simulink model "robot1v2"  (R2015a)
settings: Solver=FixedStepDiscrete  StartTime=0.0  StopTime=5  FixedStep=0.05  RelTol=1e-3
settings Model: ExtModeTrigDuration=2  Creator=Antivariant  LastModifiedBy=Antivariant
settings SolverCC: AutoInsertRateTranBlk=on
settings OptimizationCC: OptimizeModelRefInitCode=on  LifeSpan=1
settings DebuggingCC: UnderspecifiedInitializationDetection=Classic  MergeDetectMultiDrivingBlocksExec=none
settings HardwareCC: ProdBitPerInt=16  ProdBitPerPointer=8  ProdIntDivRoundTo=Zero  ProdEndianess=LittleEndian  ProdWordSize=8  ProdHWDeviceType=Atmel->AVR
settings RTWCC: SystemTargetFile=realtime.tlc  GenerateMakefile=off  TemplateMakefile=realtime.tmf  Description=Run on Target Hardware  RTWVerbose=off
settings ERTTargetCC: CombineOutputUpdateFcns=off  ExtModeTransport=3  ExtModeMexFile=ext_serial_win32_comm_rtt  ExtModeMexArgs=0 1 9600  ERTSrcFileBannerTemplate=realtime_code_template.cgt  ERTHdrFileBannerTemplate=realtime_code_template.cgt  ERTDataSrcFileTemplate=realtime_code_template.cgt  ERTDataHdrFileTemplate=realtime_code_template.cgt  ERTCustomFileTemplate=realtime_file_process.tlc

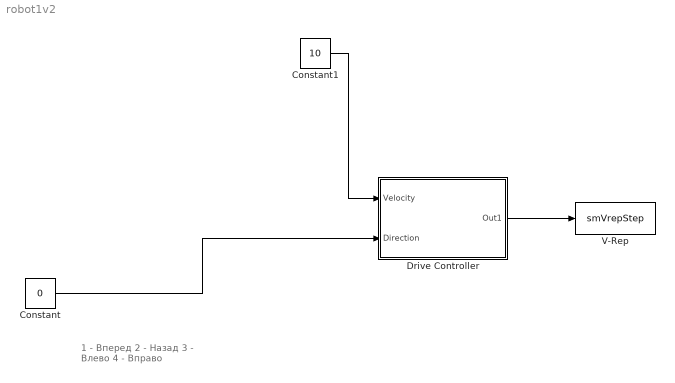
== system robot1v2 ==
  note: 1 - Вперед
      | 2 - Назад
      | 3 - Влево
      | 4 - Вправо
  Constant : Constant  Value=0  OutDataTypeStr=int8
  Constant1 : Constant  Value=10
  Drive Controller : Subsystem
      mask Display:
      | image('wheel.jpg')
      | port_label('input',1,'Velovity')
      | port_label('input',2,'Direction')
  V-Rep : M-S-Function  FunctionName=smVrepStep  Parameters=addr,port  mask{addr='127.0.0.1', port=19997}
      mask Display:
      | port_label('input',1,'in')
      | disp('V-Rep Step')
  wires:
  Constant1/1 -> Drive Controller/1(Velocity)
  Constant/1 -> Drive Controller/2(Direction)
  Drive Controller/1(Out1) -> V-Rep/1

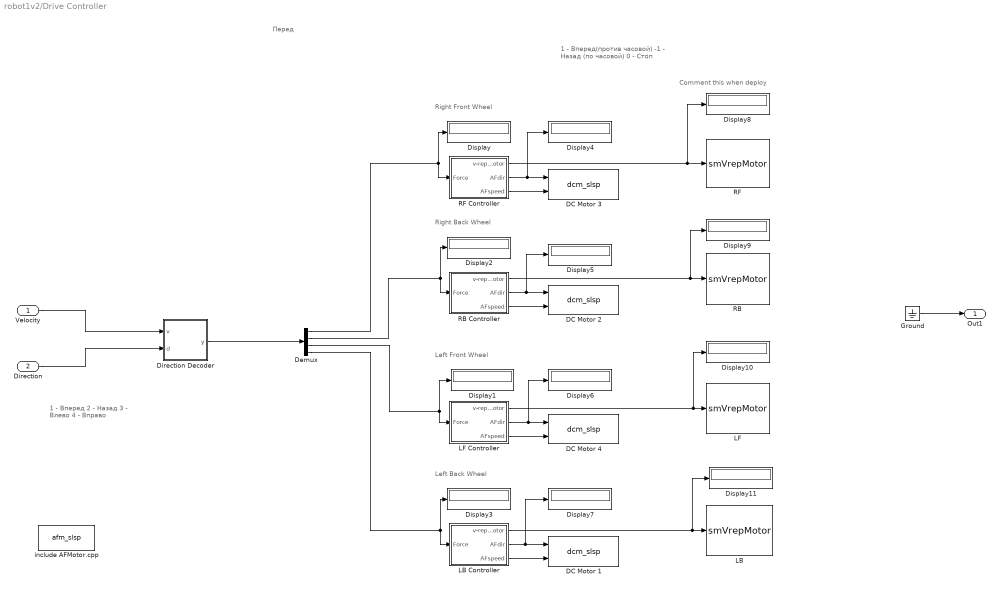
== system robot1v2/Drive Controller ==
  note: Перед
  note: 1 - Вперед
      | 2 - Назад
      | 3 - Влево
      | 4 - Вправо
  note: 1 - Вперед(против часовой)
      | -1 - Назад (по часовой)
      | 0 - Стоп
  note: Comment this when deploy
  note: Right Front Wheel
  note: Left Front Wheel
  note: Right Back Wheel
  note: Left Back Wheel
  Velocity : Inport
  Direction : Inport  Port=2
  DC Motor 1 : S-Function  InitFcn=try, set_param(gcb,'FunctionName','dcm_slsp'), end  FunctionName=dcm_slsp  Parameters=uint8(1)  SFunctionModules=dcm_slsp_wrapper  mask(S-Function Builder){}
      mask init:
      | val = [[.9  0.75 0.75 1 1 .9 .9 1]',[1 1 0.75 0.75 .9 .9 1 .9]'];try , sys = get_param(gcb,'SfunBuilderFcnName');if isempty(sys), sys = get_param(gcb,'FunctionName'); end,catch, sys = get_param(gcb,'FunctionName'); end
      settings: CopyFcn=set_param(gcbh,'LinkStatus','none')  PreSaveFcn=try, set_param(gcb,'FunctionName','dcm_slsp'), end  OpenFcn=sfunctionwizard(gcbh)
      mask Display: plot(val(:,1),val(:,2)),disp(sys), port_label('input',1,'dir'), port_label('input',2,'spd')
  DC Motor 2 : S-Function  InitFcn=try, set_param(gcb,'FunctionName','dcm_slsp'), end  FunctionName=dcm_slsp  Parameters=uint8(2)  SFunctionModules=dcm_slsp_wrapper  mask(S-Function Builder){}
      mask init: same as robot1v2/Drive Controller/DC Motor 1
      settings: CopyFcn=set_param(gcbh,'LinkStatus','none')  PreSaveFcn=try, set_param(gcb,'FunctionName','dcm_slsp'), end  OpenFcn=sfunctionwizard(gcbh)
      mask Display: plot(val(:,1),val(:,2)),disp(sys), port_label('input',1,'dir'), port_label('input',2,'spd')
  DC Motor 3 : S-Function  InitFcn=try, set_param(gcb,'FunctionName','dcm_slsp'), end  FunctionName=dcm_slsp  Parameters=uint8(3)  SFunctionModules=dcm_slsp_wrapper  mask(S-Function Builder){}
      mask init: same as robot1v2/Drive Controller/DC Motor 1
      settings: CopyFcn=set_param(gcbh,'LinkStatus','none')  PreSaveFcn=try, set_param(gcb,'FunctionName','dcm_slsp'), end  OpenFcn=sfunctionwizard(gcbh)
      mask Display: plot(val(:,1),val(:,2)),disp(sys), port_label('input',1,'dir'), port_label('input',2,'spd')
  DC Motor 4 : S-Function  InitFcn=try, set_param(gcb,'FunctionName','dcm_slsp'), end  FunctionName=dcm_slsp  Parameters=uint8(4)  SFunctionModules=dcm_slsp_wrapper  mask(S-Function Builder){}
      mask init: same as robot1v2/Drive Controller/DC Motor 1
      settings: CopyFcn=set_param(gcbh,'LinkStatus','none')  PreSaveFcn=try, set_param(gcb,'FunctionName','dcm_slsp'), end  OpenFcn=sfunctionwizard(gcbh)
      mask Display: plot(val(:,1),val(:,2)),disp(sys), port_label('input',1,'dir'), port_label('input',2,'spd')
  Demux : Demux
  Direction Decoder : Stateflow chart  TreatAsAtomicUnit=on
  Display{,1..11} (12 alike) : Display
  Ground : Ground
  LB : M-S-Function  FunctionName=smVrepMotor  Parameters=addr, port, jname  mask{addr='127.0.0.1', port=19997, jname='joint_back_left_wheel'}
      mask prompts: addr "V-Rep Server Address"; port "V-Rep Server Port"; jname "Joint name"
      mask Display:
      | image('joint.png')
      | port_label('input',1,'vel')
  LB Controller : Subsystem
  LF : M-S-Function  FunctionName=smVrepMotor  Parameters=addr, port, jname  mask{addr='127.0.0.1', port=19997, jname='joint_front_left_wheel'}
      mask prompts: addr "V-Rep Server Address"; port "V-Rep Server Port"; jname "Joint name"
      mask Display:
      | image('joint.png')
      | port_label('input',1,'vel')
  LF Controller : Subsystem
  RB : M-S-Function  FunctionName=smVrepMotor  Parameters=addr, port, jname  mask{addr='127.0.0.1', port=19997, jname='joint_back_right_wheel'}
      mask prompts: addr "V-Rep Server Address"; port "V-Rep Server Port"; jname "Joint name"
      mask Display:
      | image('joint.png')
      | port_label('input',1,'vel')
  RB Controller : Subsystem
  RF : M-S-Function  FunctionName=smVrepMotor  Parameters=addr, port, jname  mask{addr='127.0.0.1', port=19997, jname='joint_front_right_wheel'}
      mask prompts: addr "V-Rep Server Address"; port "V-Rep Server Port"; jname "Joint name"
      mask Display:
      | image('joint.png')
      | port_label('input',1,'vel')
  RF Controller : Subsystem
  include AFMotor.cpp : S-Function  InitFcn=try, set_param(gcb,'FunctionName','afm_slsp'), end  FunctionName=afm_slsp  SFunctionModules=afm_slsp_wrapper  mask(S-Function Builder){}
      mask help: Simulink:masks:SFunctionBuilder_MD
      mask init: same as robot1v2/Drive Controller/DC Motor 1
      settings: CopyFcn=set_param(gcbh,'LinkStatus','none')  PreSaveFcn=try, set_param(gcb,'FunctionName','afm_slsp'), end  OpenFcn=sfunctionwizard(gcbh)
      mask Display:
      | plot(val(:,1),val(:,2))
      | disp(sys)
  Out1 : Outport
  wires:
  LF Controller/2(AFdir) -> Display6/1, DC Motor 4/1
  Demux/3 -> Display1/1, LF Controller/1(Force)
  Demux/2 -> Display2/1, RB Controller/1(Force)
  Demux/4 -> Display3/1, LB Controller/1(Force)
  RF Controller/3(AFspeed) -> DC Motor 3/2
  LF Controller/1(v-rep motor) -> Display10/1, LF/1
  RF Controller/2(AFdir) -> Display4/1, DC Motor 3/1
  Direction Decoder/1(y) -> Demux/1
  Direction/1 -> Direction Decoder/2(d)
  Velocity/1 -> Direction Decoder/1(v)
  RF Controller/1(v-rep motor) -> Display8/1, RF/1
  LB Controller/2(AFdir) -> Display7/1, DC Motor 1/1
  RB Controller/3(AFspeed) -> DC Motor 2/2
  LB Controller/3(AFspeed) -> DC Motor 1/2
  RB Controller/2(AFdir) -> Display5/1, DC Motor 2/1
  LB Controller/1(v-rep motor) -> Display11/1, LB/1
  LF Controller/3(AFspeed) -> DC Motor 4/2
  Demux/1 -> Display/1, RF Controller/1(Force)
  RB Controller/1(v-rep motor) -> Display9/1, RB/1
  Ground/1 -> Out1/1

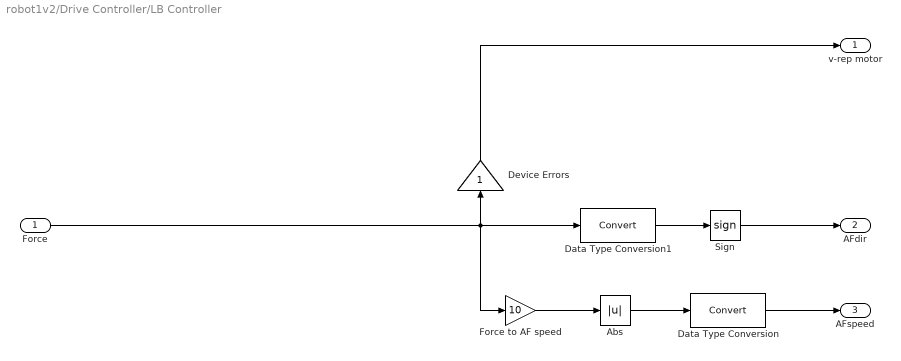
== system robot1v2/Drive Controller/LB Controller ==
  Force : Inport
  Abs : Abs
  Data Type Conversion : DataTypeConversion
  Data Type Conversion1 : DataTypeConversion
  Device Errors : Gain
  Force to AF speed : Gain  Gain=10
  Sign : Signum
  v-rep motor : Outport
  AFdir : Outport  Port=2
  AFspeed : Outport  Port=3
  wires:
  Abs/1 -> Data Type Conversion/1
  Force/1 -> Data Type Conversion1/1, Device Errors/1, Force to AF speed/1
  Force to AF speed/1 -> Abs/1
  Data Type Conversion/1 -> AFspeed/1
  Data Type Conversion1/1 -> Sign/1
  Sign/1 -> AFdir/1
  Device Errors/1 -> v-rep motor/1

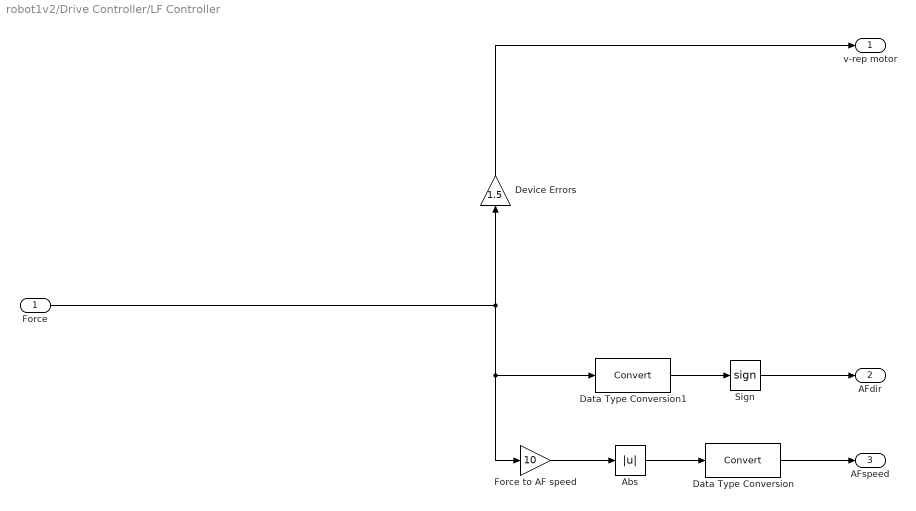
== system robot1v2/Drive Controller/LF Controller ==
  Force : Inport
  Abs : Abs
  Data Type Conversion : DataTypeConversion
  Data Type Conversion1 : DataTypeConversion
  Device Errors : Gain  Gain=1.5
  Force to AF speed : Gain  Gain=10
  Sign : Signum
  v-rep motor : Outport
  AFdir : Outport  Port=2
  AFspeed : Outport  Port=3
  wires:
  Abs/1 -> Data Type Conversion/1
  Force to AF speed/1 -> Abs/1
  Data Type Conversion/1 -> AFspeed/1
  Force/1 -> Device Errors/1, Data Type Conversion1/1, Force to AF speed/1
  Data Type Conversion1/1 -> Sign/1
  Sign/1 -> AFdir/1
  Device Errors/1 -> v-rep motor/1

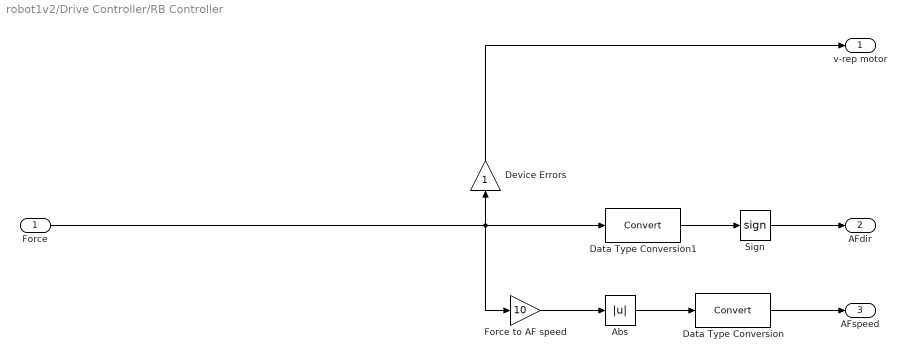
== system robot1v2/Drive Controller/RB Controller ==
  Force : Inport
  Abs : Abs
  Data Type Conversion : DataTypeConversion
  Data Type Conversion1 : DataTypeConversion
  Device Errors : Gain
  Force to AF speed : Gain  Gain=10
  Sign : Signum
  v-rep motor : Outport
  AFdir : Outport  Port=2
  AFspeed : Outport  Port=3
  wires:
  Data Type Conversion/1 -> AFspeed/1
  Force to AF speed/1 -> Abs/1
  Force/1 -> Data Type Conversion1/1, Device Errors/1, Force to AF speed/1
  Abs/1 -> Data Type Conversion/1
  Data Type Conversion1/1 -> Sign/1
  Sign/1 -> AFdir/1
  Device Errors/1 -> v-rep motor/1

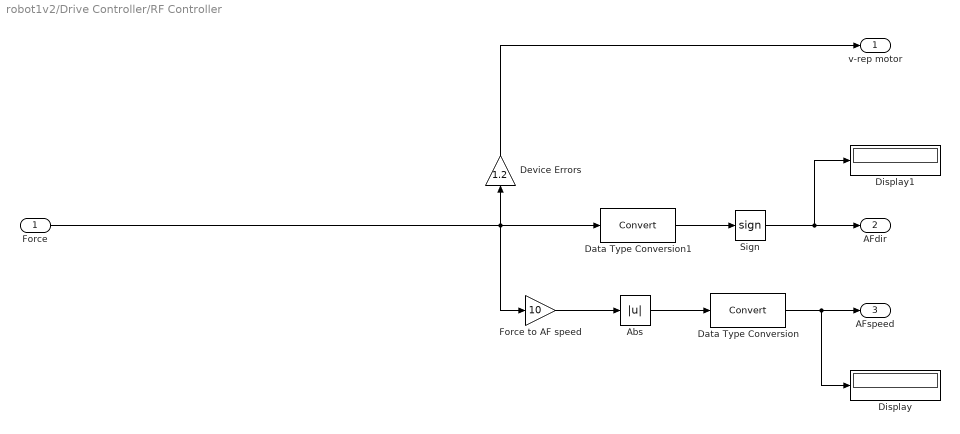
== system robot1v2/Drive Controller/RF Controller ==
  Force : Inport
  Abs : Abs
  Data Type Conversion : DataTypeConversion
  Data Type Conversion1 : DataTypeConversion
  Device Errors : Gain  Gain=1.2
  Display : Display
  Display1 : Display
  Force to AF speed : Gain  Gain=10
  Sign : Signum
  v-rep motor : Outport
  AFdir : Outport  Port=2
  AFspeed : Outport  Port=3
  wires:
  Data Type Conversion/1 -> Display/1, AFspeed/1
  Force to AF speed/1 -> Abs/1
  Force/1 -> Data Type Conversion1/1, Device Errors/1, Force to AF speed/1
  Abs/1 -> Data Type Conversion/1
  Sign/1 -> Display1/1, AFdir/1
  Data Type Conversion1/1 -> Sign/1
  Device Errors/1 -> v-rep motor/1

== stateflow chart robot1v2/Drive Controller/Direction Decoder ==
  state Stop
    entry: y=[0 0 0 0]
  state Forward
    entry: y=[-v -v v v];
  state Backward
    entry: y=[v v -v -v];
  state Left
    entry: y=[-v -v -v -v];
  state Right
    entry: y=[v v v v];
  (default) -> Stop
  Stop -> Forward [order 1] : [d==1]
  Stop -> Right [order 4] : [d==4]
  Stop -> Left [order 3] : [d==3]
  Stop -> Backward [order 2] : [d==2]
  data: v input; y output; d input
